simulink model "SIMULINK_ADP_Tracking"  (R2023b)
settings: Solver=FixedStepAuto  StartTime=0.0  StopTime=sim_end_time  FixedStep=fixed_step_size  RelTol=1e-3
undefined symbols (not defined in the file): a, act_end, b, battery_threshold, bb, delta_, draw_gif, droneyeeUAV2_NUM, droneyeeUAV3_NUM, droneyeeUAV4_NUM, droneyeeUAV5_NUM, fixed_step_size, k, KD_x, KD_y, kd_z, KDD_x, KDD_y, KI_x, KI_y, ki_z, KII_x, KII_y, KP_x, KP_y, kp_z, KPP_x, KPP_y, lmt, omega, omega_, R, sim_end_time, uav10num, uav1num, uav2num, uav3num, uav4num, uav5num, uav6num, uav7num, uav8num, uav9num, UAV_NUM, Vel_Switch_1, Vel_Switch_10, Vel_Switch_11, Vel_Switch_12, Vel_Switch_13, Vel_Switch_14, Vel_Switch_15, Vel_Switch_16, Vel_Switch_17, Vel_Switch_18, Vel_Switch_19, Vel_Switch_2, Vel_Switch_20, Vel_Switch_3, Vel_Switch_4, Vel_Switch_5 ... (+16)
libraries: simulink x118, aerolibanimutils x1
(part 1 of 11)
settings Model: Creator=exbot  LastModifiedBy=tanju
settings SolverCC: AlgebraicLoopSolver=TrustRegion
settings DataIOCC: LimitDataPoints=on  ReturnWorkspaceOutputs=off
settings OptimizationCC: DefaultParameterBehavior=Inlined  ReuseModelBlockBuffer=off  PassReuseOutputArgsAs=Individual arguments  MaxStackSize=64  EfficientTunableParamExpr=on
settings DebuggingCC: ParameterTunabilityLossMsg=error  UnconnectedInputMsg=warning  UnconnectedOutputMsg=warning  UnconnectedLineMsg=warning  AllowSymbolicDim=off  SFUnexpectedBacktrackingDiag=warning  SFNoUnconditionalDefaultTransitionDiag=warning  SFExecutionAtInitializationDiag=none  ArithmeticOperatorsInVariantConditions=warning
settings HardwareCC: ProdBitPerPointer=32  ProdBitPerSizeT=32  ProdBitPerPtrDiffT=32  ProdLargestAtomicFloat=None  ProdIntDivRoundTo=Undefined  ProdEndianess=Unspecified  ProdWordSize=32  ProdHWDeviceType=Generic->Unspecified (assume 32-bit Generic)  TargetBitPerPointer=64  TargetBitPerSizeT=64  TargetBitPerPtrDiffT=64  TargetLongLongMode=on  TargetIntDivRoundTo=Zero  TargetEndianess=LittleEndian  TargetWordSize=64  TargetHWDeviceType=MATLAB Host  ProdEqTarget=off
settings ModelReferenceCC: EnableRefExpFcnMdlSchedulingChecks=on  PropagateSignalLabelsOutOfModel=off
settings SFSimCC: SimUseLocalCustomCode=off  MATLABDynamicMemAlloc=off  CustomCodeUndefinedFunction=UseInterfaceOnly
settings RTWCC: Description=Embedded Coder (host-based shared library target)  SystemTargetFile=ert_shrlib.tlc  TemplateMakefile=ert_default_tmf  GenerateReport=on  RTWUseLocalCustomCode=off  IncludeHyperlinkInReport=on  LaunchReport=on  GenerateTraceInfo=on  GenerateTraceReport=on  GenerateTraceReportSl=on  GenerateTraceReportSf=on  GenerateTraceReportEml=on
settings CodeAppCC: ForceParamTrailComments=on  IgnoreCustomStorageClasses=off  OperatorAnnotations=on  SimulinkDataObjDesc=on  SFDataObjDesc=on  InsertBlockDesc=on
settings STFCustomTargetCC: TargetLangStandard=C89/C90 (ANSI)  MultiwordLength=256  GenerateSampleERTMain=on  ParMdlRefBuildCompliant=on  CompOptLevelCompliant=on  CombineOutputUpdateFcns=on  ERTCustomFileBanners=on  RemoveResetFunc=on  MATLABClassNameForMDSCustomization=Simulink.SoftwareTarget.ERTCustomization  ModelStepFunctionPrototypeControlCompliant=on  UseToolchainInfoCompliant=on  SystemTargetFile=ert_shrlib.tlc
settings ERTTargetCC: GenerateSampleERTMain=on  ConcurrentExecutionCompliant=off  SupportContinuousTime=on  SupportNonInlinedSFcns=on  CPPClassGenCompliant=off  InlinedParameterPlacement=NonHierarchical  ERTCustomFileTemplate=example_file_process.tlc
settings ConfigComp: CovMetricSettings=dw  CovSaveCumulativeToWorkspaceVar=on  CovSaveSingleToWorkspaceVar=on  CovExternalEMLEnable=off

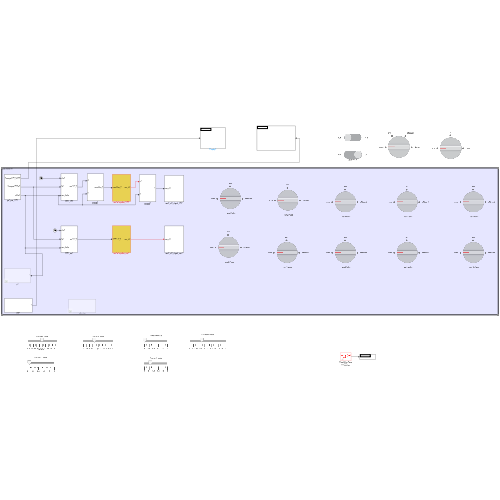
[thumbnail: Simulink's stored preview of the top-level diagram]
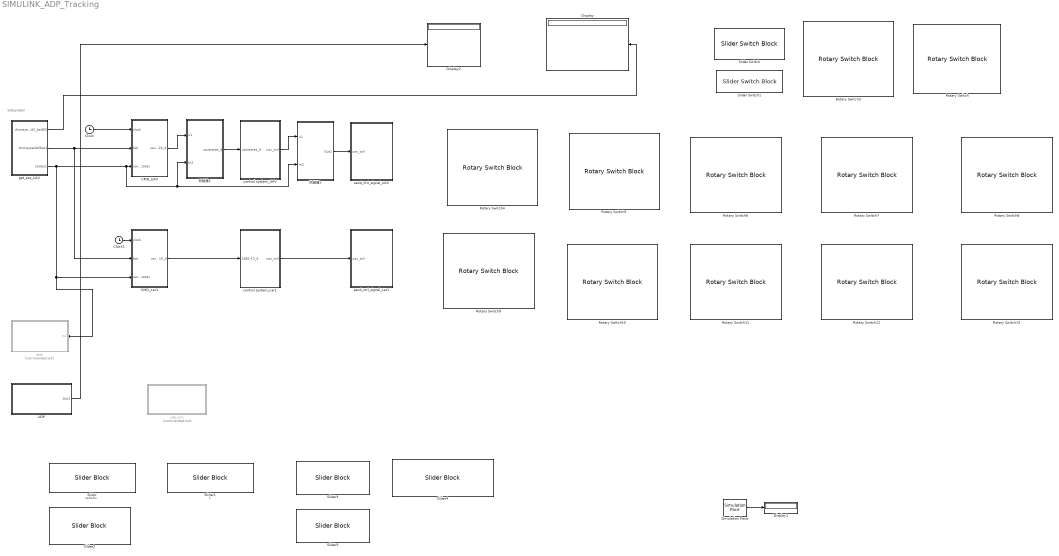
== system SIMULINK_ADP_Tracking ==
  note: Subsystem
  note: safedis
  note: k
  CMD_UAV : Subsystem
  CMD_car1 : Subsystem
  Clock : Clock
  Clock1 : Clock
  Display : Display
  Display1 : Display
  Display2 : Display
  Rotary Switch : RotarySwitchBlock  LabelPosition=Hide
      settings: Values={{'land', 'trj', 'hover'}, [-1 2 1]}
  Rotary Switch{4..13} (10 alike) : RotarySwitchBlock  LabelPosition=Bottom
      settings: Values={{'none', 'arm', 'offboard'}, [0 2 3]}
  Rotary Switch3 : RotarySwitchBlock  LabelPosition=Hide
      settings: Values={{'none', 'arm', 'offboard', 'disram'}, [0 2 3 5]}
  Simulation Pace : aerolibanimutils/Simulation Pace  SimulationPace=1  SleepMode=MATLAB Thread  OutputPaceError=on  SampleTime=-1
  Slider{,2..5} (5 alike) : SliderBlock  ScaleMax=2
  Slider Switch : SliderSwitchBlock  LabelPosition=Hide
      settings: Values={{'仿真', '实飞'}, [-1 1]}
  Slider Switch1 : SliderSwitchBlock  LabelPosition=Bottom
      settings: Values={{'Off', 'On'}, [0 1]}
  Slider1 : SliderBlock  ScaleMax=5
  UDP : Subsystem
  control system_UAV : Subsystem
  control system_car1 : Subsystem
  get_pos_UAV : Subsystem
  plot : Subsystem  Commented=on
  send_ctrl_signal_UAV : Subsystem
  send_ctrl_signal_car1 : Subsystem
  udp_sim : Subsystem  Commented=on
  防碰撞1 : Subsystem
  防碰撞2 : Subsystem
  wires:
  Simulation Pace/1 -> Display1/1
  UDP/1(Out1) -> Display2/1
  get_pos_UAV/1(droneyeeUAV_batDIS) -> Display/1
  防碰撞1/1(uavstates_d) -> control system_UAV/1(uavstates_d)
  CMD_UAV/1(uav1-24_d) -> 防碰撞1/1(u1)
  control system_UAV/1(uav_ctrl) -> 防碰撞2/1(u1)
  防碰撞2/1(Out1) -> send_ctrl_signal_UAV/1(uav_ctrl)
  Clock1/1 -> CMD_car1/1(clock)
  get_pos_UAV/3(states1) -> CMD_car1/3(uav_states), plot/1(In1), 防碰撞2/2(In2), 防碰撞1/2(In2), CMD_UAV/3(uav_states)
  Clock/1 -> CMD_UAV/1(clock)
  get_pos_UAV/2(droneyeeUAVbat1) -> CMD_car1/2(bat), CMD_UAV/2(bat)
  control system_car1/1(uav_ctrl) -> send_ctrl_signal_car1/1(uav_ctrl)
  CMD_car1/1(car1-10_d) -> control system_car1/1(CAR1-10_d)

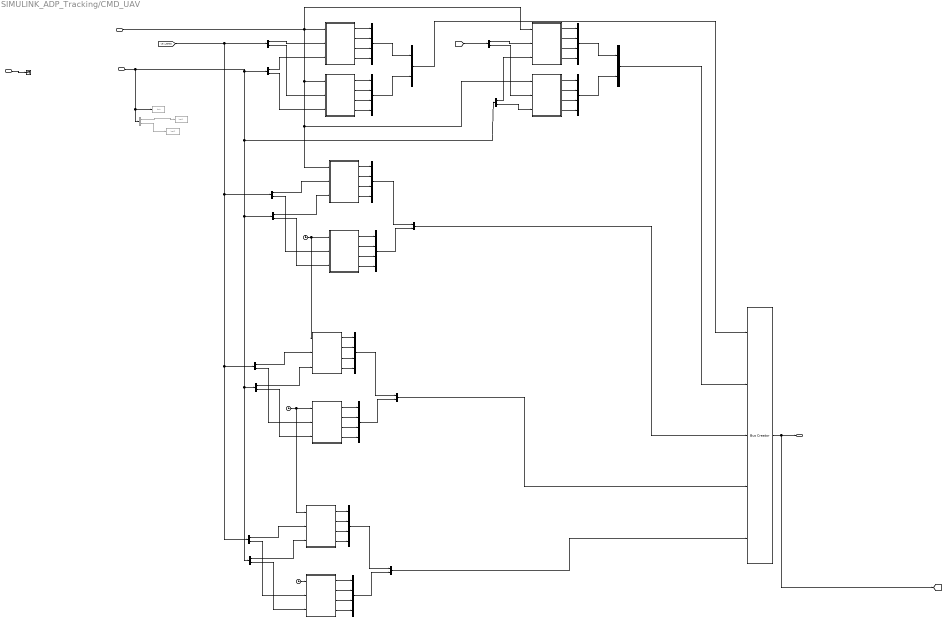
== system SIMULINK_ADP_Tracking/CMD_UAV ==
  clock : Inport
  bat : Inport  Port=2
  uav_states : Inport  Port=3
  Bus Creator{,1,3..4,6..7,9..10,12..13} (10 alike) : BusCreator  Inputs=4
  Bus Creator{2,5,8,11,14} (5 alike) : BusCreator  Inputs=2
  Bus Creator36 : BusCreator  Inputs=5
  Bus Selector : BusSelector  OutputSignals=droneyeeUAV1bat,droneyeeUAV2bat
  Bus Selector1 : BusSelector  OutputSignals=droneyeeUAV1_states,droneyeeUAV2_states
  Bus Selector10 : BusSelector  OutputSignals=droneyeeUAV9bat,droneyeeUAV10bat
  Bus Selector2 : BusSelector  OutputSignals=droneyeeUAV5_states,droneyeeUAV6_states
  Bus Selector3 : BusSelector  OutputSignals=droneyeeUAV3_states,droneyeeUAV4_states
  Bus Selector4 : BusSelector  OutputSignals=droneyeeUAV3bat,droneyeeUAV4bat
  Bus Selector5 : BusSelector  OutputSignals=droneyeeUAV5bat,droneyeeUAV6bat
  Bus Selector6 : BusSelector  Commented=on  OutputSignals=droneyeeUAV1bat,droneyeeUAV2bat
  Bus Selector7 : BusSelector  OutputSignals=droneyeeUAV7_states,droneyeeUAV8_states
  Bus Selector8 : BusSelector  OutputSignals=droneyeeUAV7bat,droneyeeUAV8bat
  Bus Selector9 : BusSelector  OutputSignals=droneyeeUAV9_states,droneyeeUAV10_states
  CMD1 : Subsystem
  CMD10 : Subsystem
  CMD2 : Subsystem
  CMD3 : Subsystem
  CMD4 : Subsystem
  CMD5 : Subsystem
  CMD6 : Subsystem
  CMD7 : Subsystem
  CMD8 : Subsystem
  CMD9 : Subsystem
  Clock : Clock
  Clock1 : Clock
  Clock2 : Clock
  Terminator : Terminator
  To Workspace : ToWorkspace  Commented=on  VariableName=bat  SampleTime=-1
  To Workspace1 : ToWorkspace  Commented=on  VariableName=bat1  SampleTime=-1
  To Workspace2 : ToWorkspace  Commented=on  VariableName=bat2  SampleTime=-1
  uav1-24_d : Outport  VectorParamsAs1DForOutWhenUnconnected=off
  tag scope: uav1_24_d1=global
  wires:
  CMD1/1(x_d) -> Bus Creator/1  "x1_d"
  CMD1/2(y_d) -> Bus Creator/2  "y1_d"
  CMD1/3(z_d) -> Bus Creator/3  "z1_d"
  CMD1/4(yaw_d) -> Bus Creator/4  "yaw1_d"
  CMD2/1(x_d) -> Bus Creator1/1  "x2_d"
  CMD2/2(y_d) -> Bus Creator1/2  "y2_d"
  CMD2/3(z_d) -> Bus Creator1/3  "z2_d"
  CMD2/4(yaw_d) -> Bus Creator1/4  "yaw2_d"
  Bus Creator/1 -> Bus Creator2/1  "droneyeeUAV1_d"
  Bus Creator1/1 -> Bus Creator2/2  "droneyeeUAV2_d"
  Bus Creator2/1 -> Bus Creator36/1  "states1_2_d"
  Bus Creator3/1 -> Bus Creator5/1  "droneyeeUAV3_d"
  Bus Creator4/1 -> Bus Creator5/2  "droneyeeUAV4_d"
  CMD3/2(y_d) -> Bus Creator3/2  "y3_d"
  CMD3/3(z_d) -> Bus Creator3/3  "z3_d"
  CMD3/4(yaw_d) -> Bus Creator3/4  "yaw3_d"
  Bus Creator5/1 -> Bus Creator36/2  "states_3_4_d"
  CMD4/1(x_d) -> Bus Creator4/1  "x4_d"
  CMD3/1(x_d) -> Bus Creator3/1  "x3_d"
  CMD4/2(y_d) -> Bus Creator4/2  "y4_d"
  CMD4/4(yaw_d) -> Bus Creator4/4  "yaw4_d"
  CMD4/3(z_d) -> Bus Creator4/3  "z4_d"
  CMD5/2(y_d) -> Bus Creator6/2  "y5_d"
  CMD5/3(z_d) -> Bus Creator6/3  "z5_d"
  CMD5/4(yaw_d) -> Bus Creator6/4  "yaw5_d"
  CMD5/1(x_d) -> Bus Creator6/1  "x5_d"
  Bus Creator8/1 -> Bus Creator36/3  "states_5_6_d"
  Bus Selector1/1 -> CMD1/2(droneyeeUAV_states)  "<droneyeeUAV1_states>"
  Bus Selector1/2 -> CMD2/2(droneyeeUAV_states)  "<droneyeeUAV2_states>"
  Bus Selector/1 -> CMD1/3(droneyeeUAV_bat)  "<droneyeeUAV1bat>"
  Bus Selector/2 -> CMD2/3(droneyeeUAV_bat)  "<droneyeeUAV2bat>"
  Bus Selector2/1 -> CMD5/2(droneyeeUAV_states)  "<droneyeeUAV5_states>"
  [uav_states] -> Bus Selector3/1
  Bus Selector3/1 -> CMD3/2(droneyeeUAV_states)  "<droneyeeUAV3_states>"
  Bus Selector3/2 -> CMD4/2(droneyeeUAV_states)  "<droneyeeUAV4_states>"
  Bus Selector4/1 -> CMD3/3(droneyeeUAV_bat)  "<droneyeeUAV3bat>"
  Bus Selector4/2 -> CMD4/3(droneyeeUAV_bat)  "<droneyeeUAV4bat>"
  Bus Selector5/1 -> CMD5/3(droneyeeUAV_bat)  "<droneyeeUAV5bat>"
  clock/1 -> CMD3/1("clock "), CMD2/1("clock "), CMD4/1("clock "), CMD5/1("clock "), CMD1/1("clock ")
  Bus Creator36/1 -> [uav1_24_d1], uav1-24_d/1
  uav_states/1 -> Terminator/1
  Bus Selector6/1 -> To Workspace1/1  "<droneyeeUAV1bat>"
  Bus Selector6/2 -> To Workspace2/1  "<droneyeeUAV2bat>"
  CMD6/2(y_d) -> Bus Creator7/2  "y1_d"
  CMD6/1(x_d) -> Bus Creator7/1  "x1_d"
  CMD6/3(z_d) -> Bus Creator7/3  "z1_d"
  CMD6/4(yaw_d) -> Bus Creator7/4  "yaw1_d"
  Bus Selector5/2 -> CMD6/3(droneyeeUAV_bat)  "<droneyeeUAV6bat>"
  Bus Selector2/2 -> CMD6/2(droneyeeUAV_states)  "<droneyeeUAV6_states>"
  Bus Creator6/1 -> Bus Creator8/1  "droneyeeUAV5_d"
  Bus Creator7/1 -> Bus Creator8/2  "droneyeeUAV4_d"
  Bus Creator10/1 -> Bus Creator11/2  "droneyeeUAV4_d"
  Clock/1 -> CMD7/1("clock "), CMD6/1("clock ")
  CMD7/1(x_d) -> Bus Creator9/1  "x5_d"
  Bus Creator9/1 -> Bus Creator11/1  "droneyeeUAV5_d"
  Bus Selector7/1 -> CMD7/2(droneyeeUAV_states)  "<droneyeeUAV7_states>"
  CMD7/4(yaw_d) -> Bus Creator9/4  "yaw5_d"
  Bus Selector8/1 -> CMD7/3(droneyeeUAV_bat)  "<droneyeeUAV7bat>"
  CMD7/2(y_d) -> Bus Creator9/2  "y5_d"
  CMD7/3(z_d) -> Bus Creator9/3  "z5_d"
  CMD8/2(y_d) -> Bus Creator10/2  "y1_d"
  CMD8/3(z_d) -> Bus Creator10/3  "z1_d"
  CMD8/1(x_d) -> Bus Creator10/1  "x1_d"
  Bus Selector8/2 -> CMD8/3(droneyeeUAV_bat)  "<droneyeeUAV8bat>"
  Bus Selector7/2 -> CMD8/2(droneyeeUAV_states)  "<droneyeeUAV8_states>"
  CMD8/4(yaw_d) -> Bus Creator10/4  "yaw1_d"
  Bus Creator13/1 -> Bus Creator14/2  "droneyeeUAV4_d"
  Clock1/1 -> CMD8/1("clock "), CMD9/1("clock ")
  CMD9/1(x_d) -> Bus Creator12/1  "x5_d"
  Bus Creator12/1 -> Bus Creator14/1  "droneyeeUAV5_d"
  bat/1 -> Bus Selector6/1, To Workspace/1, Bus Selector10/1, Bus Selector8/1, Bus Selector5/1, Bus Selector4/1, Bus Selector/1
  Bus Selector9/1 -> CMD9/2(droneyeeUAV_states)  "<droneyeeUAV9_states>"
  CMD9/4(yaw_d) -> Bus Creator12/4  "yaw5_d"
  [uav_states] -> Bus Selector9/1, Bus Selector7/1, Bus Selector2/1, Bus Selector1/1
  Bus Selector10/1 -> CMD9/3(droneyeeUAV_bat)  "<droneyeeUAV9bat>"
  CMD9/2(y_d) -> Bus Creator12/2  "y5_d"
  CMD9/3(z_d) -> Bus Creator12/3  "z5_d"
  CMD10/2(y_d) -> Bus Creator13/2  "y1_d"
  CMD10/3(z_d) -> Bus Creator13/3  "z1_d"
  CMD10/1(x_d) -> Bus Creator13/1  "x1_d"
  Bus Selector10/2 -> CMD10/3(droneyeeUAV_bat)  "<droneyeeUAV10bat>"
  Clock2/1 -> CMD10/1("clock ")
  Bus Selector9/2 -> CMD10/2(droneyeeUAV_states)  "<droneyeeUAV10_states>"
  CMD10/4(yaw_d) -> Bus Creator13/4  "yaw1_d"
  Bus Creator11/1 -> Bus Creator36/4  "states_7_8_d"
  Bus Creator14/1 -> Bus Creator36/5  "states_9_10_d"

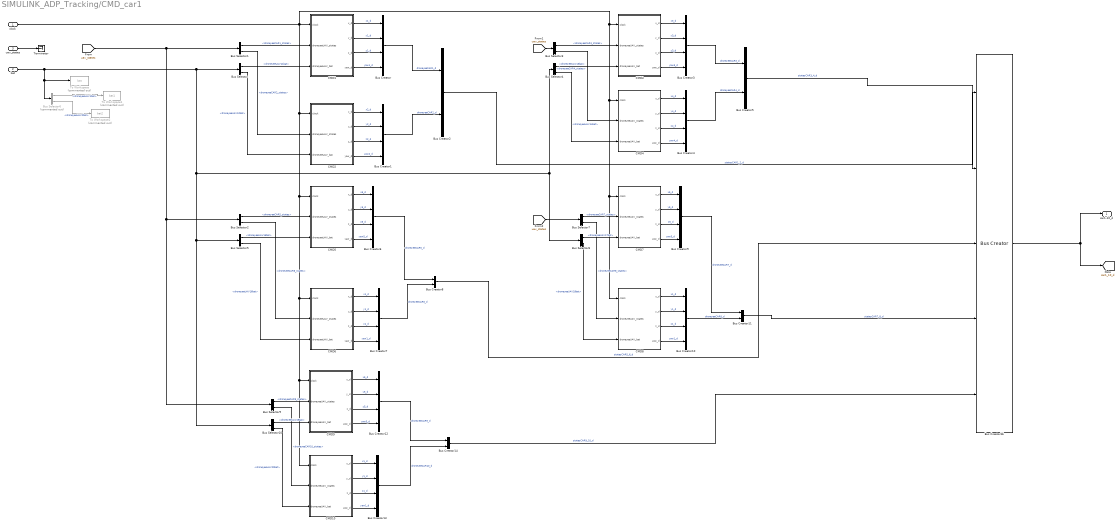
== system SIMULINK_ADP_Tracking/CMD_car1 ==
  clock : Inport
  bat : Inport  Port=2
  uav_states : Inport  Port=3
  Bus Creator{,1,3..4,6..7,9..10,12..13} (10 alike) : BusCreator  Inputs=4
  Bus Creator{2,5,8,11,14} (5 alike) : BusCreator  Inputs=2
  Bus Creator36 : BusCreator  Inputs=5
  Bus Selector : BusSelector  OutputSignals=droneyeeUAV11bat,droneyeeUAV12bat
  Bus Selector1 : BusSelector  OutputSignals=droneyeeCAR1_states,droneyeeCAR2_states
  Bus Selector10 : BusSelector  OutputSignals=droneyeeUAV19bat,droneyeeUAV20bat
  Bus Selector2 : BusSelector  OutputSignals=droneyeeCAR5_states,droneyeeCAR6_states
  Bus Selector3 : BusSelector  OutputSignals=droneyeeCAR3_states,droneyeeCAR4_states
  Bus Selector4 : BusSelector  OutputSignals=droneyeeUAV13bat,droneyeeUAV14bat
  Bus Selector5 : BusSelector  OutputSignals=droneyeeUAV15bat,droneyeeUAV16bat
  Bus Selector6 : BusSelector  Commented=on  OutputSignals=droneyeeUAV1bat,droneyeeUAV2bat
  Bus Selector7 : BusSelector  OutputSignals=droneyeeCAR7_states,droneyeeCAR8_states
  Bus Selector8 : BusSelector  OutputSignals=droneyeeUAV17bat,droneyeeUAV18bat
  Bus Selector9 : BusSelector  OutputSignals=droneyeeCAR9_states,droneyeeCAR10_states
  CMD1 : Subsystem
  CMD10 : Subsystem
  CMD2 : Subsystem
  CMD3 : Subsystem
  CMD4 : Subsystem
  CMD5 : Subsystem
  CMD6 : Subsystem
  CMD7 : Subsystem
  CMD8 : Subsystem
  CMD9 : Subsystem
  Terminator : Terminator
  To Workspace : ToWorkspace  Commented=on  VariableName=bat  SampleTime=-1
  To Workspace1 : ToWorkspace  Commented=on  VariableName=bat1  SampleTime=-1
  To Workspace2 : ToWorkspace  Commented=on  VariableName=bat2  SampleTime=-1
  car1-10_d : Outport  VectorParamsAs1DForOutWhenUnconnected=off
  tag scope: car1_10_d=global
  wires:
  CMD1/1(x_d) -> Bus Creator/1  "x1_d"
  CMD1/2(y_d) -> Bus Creator/2  "y1_d"
  CMD1/3(z_d) -> Bus Creator/3  "z1_d"
  CMD1/4(yaw_d) -> Bus Creator/4  "yaw1_d"
  CMD2/1(x_d) -> Bus Creator1/1  "x2_d"
  CMD2/2(y_d) -> Bus Creator1/2  "y2_d"
  CMD2/3(z_d) -> Bus Creator1/3  "z2_d"
  CMD2/4(yaw_d) -> Bus Creator1/4  "yaw2_d"
  Bus Creator/1 -> Bus Creator2/1  "droneyeeCAR1_d"
  Bus Creator1/1 -> Bus Creator2/2  "droneyeeCAR2_d"
  Bus Creator3/1 -> Bus Creator5/1  "droneyeeCAR3_d"
  Bus Creator4/1 -> Bus Creator5/2  "droneyeeCAR4_d"
  CMD3/2(y_d) -> Bus Creator3/2  "y3_d"
  CMD3/3(z_d) -> Bus Creator3/3  "z3_d"
  CMD3/4(yaw_d) -> Bus Creator3/4  "yaw3_d"
  Bus Creator5/1 -> Bus Creator36/2  "statesCAR3_4_d"
  CMD4/1(x_d) -> Bus Creator4/1  "x4_d"
  CMD3/1(x_d) -> Bus Creator3/1  "x3_d"
  CMD4/2(y_d) -> Bus Creator4/2  "y4_d"
  CMD4/4(yaw_d) -> Bus Creator4/4  "yaw4_d"
  CMD4/3(z_d) -> Bus Creator4/3  "z4_d"
  CMD5/2(y_d) -> Bus Creator6/2  "y5_d"
  CMD5/3(z_d) -> Bus Creator6/3  "z5_d"
  CMD5/4(yaw_d) -> Bus Creator6/4  "yaw5_d"
  CMD5/1(x_d) -> Bus Creator6/1  "x5_d"
  Bus Creator8/1 -> Bus Creator36/3  "statesCAR5_6_d"
  Bus Selector1/1 -> CMD1/2(droneyeeUAV_states)  "<droneyeeCAR1_states>"
  Bus Selector1/2 -> CMD2/2(droneyeeUAV_states)  "<droneyeeCAR2_states>"
  Bus Selector/1 -> CMD1/3(droneyeeUAV_bat)  "<droneyeeUAV11bat>"
  Bus Selector/2 -> CMD2/3(droneyeeUAV_bat)  "<droneyeeUAV12bat>"
  Bus Selector2/1 -> CMD5/2(droneyeeUAV_states)  "<droneyeeCAR5_states>"
  [uav_states] -> Bus Selector3/1
  Bus Selector3/1 -> CMD3/2(droneyeeUAV_states)  "<droneyeeCAR3_states>"
  Bus Selector3/2 -> CMD4/2(droneyeeUAV_states)  "<droneyeeCAR4_states>"
  Bus Selector4/1 -> CMD3/3(droneyeeUAV_bat)  "<droneyeeUAV13bat>"
  Bus Selector4/2 -> CMD4/3(droneyeeUAV_bat)  "<droneyeeUAV14bat>"
  Bus Selector5/1 -> CMD5/3(droneyeeUAV_bat)  "<droneyeeUAV15bat>"
  clock/1 -> CMD8/1("clock "), CMD7/1("clock "), CMD4/1("clock "), CMD3/1("clock "), CMD10/1("clock "), CMD9/1("clock "), CMD6/1("clock "), CMD5/1("clock "), CMD2/1("clock "), CMD1/1("clock ")
  Bus Creator36/1 -> car1-10_d/1, [car1_10_d]
  uav_states/1 -> Terminator/1
  Bus Selector6/1 -> To Workspace1/1  "<droneyeeUAV1bat>"
  Bus Selector6/2 -> To Workspace2/1  "<droneyeeUAV2bat>"
  CMD6/2(y_d) -> Bus Creator7/2  "y1_d"
  CMD6/1(x_d) -> Bus Creator7/1  "x1_d"
  CMD6/3(z_d) -> Bus Creator7/3  "z1_d"
  CMD6/4(yaw_d) -> Bus Creator7/4  "yaw1_d"
  Bus Selector5/2 -> CMD6/3(droneyeeUAV_bat)  "<droneyeeUAV16bat>"
  Bus Selector2/2 -> CMD6/2(droneyeeUAV_states)  "<droneyeeCAR6_states>"
  Bus Creator6/1 -> Bus Creator8/1  "droneyeeCAR5_d"
  Bus Creator7/1 -> Bus Creator8/2  "droneyeeCAR6_d"
  Bus Creator10/1 -> Bus Creator11/2  "droneyeeCAR8_d"
  CMD7/1(x_d) -> Bus Creator9/1  "x5_d"
  Bus Creator9/1 -> Bus Creator11/1  "droneyeeCAR7_d"
  Bus Selector7/1 -> CMD7/2(droneyeeUAV_states)  "<droneyeeCAR7_states>"
  CMD7/4(yaw_d) -> Bus Creator9/4  "yaw5_d"
  Bus Selector8/1 -> CMD7/3(droneyeeUAV_bat)  "<droneyeeUAV17bat>"
  CMD7/2(y_d) -> Bus Creator9/2  "y5_d"
  CMD7/3(z_d) -> Bus Creator9/3  "z5_d"
  CMD8/2(y_d) -> Bus Creator10/2  "y1_d"
  CMD8/3(z_d) -> Bus Creator10/3  "z1_d"
  CMD8/1(x_d) -> Bus Creator10/1  "x1_d"
  Bus Selector8/2 -> CMD8/3(droneyeeUAV_bat)  "<droneyeeUAV18bat>"
  Bus Selector7/2 -> CMD8/2(droneyeeUAV_states)  "<droneyeeCAR8_states>"
  CMD8/4(yaw_d) -> Bus Creator10/4  "yaw1_d"
  Bus Creator13/1 -> Bus Creator14/2  "droneyeeCAR10_d"
  CMD9/1(x_d) -> Bus Creator12/1  "x5_d"
  Bus Creator12/1 -> Bus Creator14/1  "droneyeeCAR9_d"
  bat/1 -> Bus Selector6/1, To Workspace/1, Bus Selector10/1, Bus Selector5/1, Bus Selector8/1, Bus Selector4/1, Bus Selector/1
  CMD9/4(yaw_d) -> Bus Creator12/4  "yaw5_d"
  [uav_states] -> Bus Selector9/1, Bus Selector2/1, Bus Selector1/1
  CMD9/2(y_d) -> Bus Creator12/2  "y5_d"
  CMD9/3(z_d) -> Bus Creator12/3  "z5_d"
  CMD10/2(y_d) -> Bus Creator13/2  "y1_d"
  CMD10/3(z_d) -> Bus Creator13/3  "z1_d"
  CMD10/1(x_d) -> Bus Creator13/1  "x1_d"
  CMD10/4(yaw_d) -> Bus Creator13/4  "yaw1_d"
  Bus Creator11/1 -> Bus Creator36/4  "statesCAR7_8_d"
  Bus Creator14/1 -> Bus Creator36/5  "statesCAR9_10_d"
  [uav_states] -> Bus Selector7/1
  Bus Selector9/1 -> CMD9/2(droneyeeUAV_states)  "<droneyeeCAR9_states>"
  Bus Selector9/2 -> CMD10/2(droneyeeUAV_states)  "<droneyeeCAR10_states>"
  Bus Selector10/1 -> CMD9/3(droneyeeUAV_bat)  "<droneyeeUAV19bat>"
  Bus Selector10/2 -> CMD10/3(droneyeeUAV_bat)  "<droneyeeUAV20bat>"
  Bus Creator2/1 -> Bus Creator36/1  "statesCAR1_2_d"

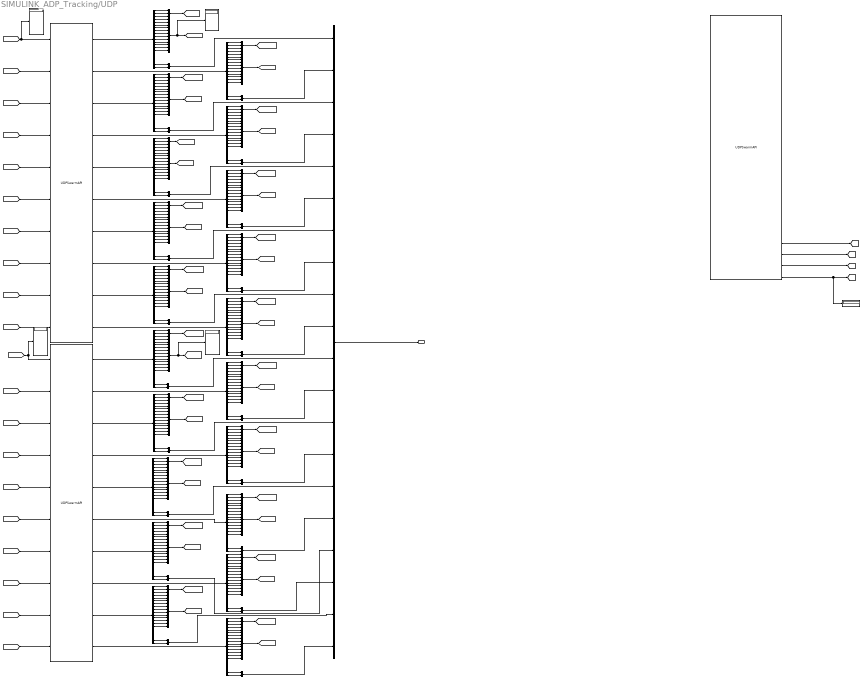
== system SIMULINK_ADP_Tracking/UDP ==
  note: 这个UDP模块的端口为 26000+(Id-1)*2
      | Simulink输入维度为0,
      | 输出维度为3，对应UDP接收的[Double bat1, Double bat2, Double bat3]
      |
      | 这个UDP模块的发送端口为 26000+(Id-1)*2+1（但是这里没有使用）
  CopterRecA : S-Function  FunctionName=UDPSwarmAPI  Parameters=port,num,modeValue,T,ip  SFunctionDeploymentMode=off  EnableBusSupport=off  mask(UDP Receive){ip=127.0.0.1, port=27000, num=10, mode=CopterRecA, T=-1, modeValue=0}
      mask prompts: ip "UDP IP Address"; port "UDP Port"; num "vehicle Number"; mode "UDP Mode"; T "Sample Time"
      mask help:
      | This block receives bytes from an UDP/IP connection.
      | The first parameter is the UDP port on the first CopterSim App
      | The second parameter is the total vehicle number
      | The third parameter is the data mode. check the help button for the definition
      mask init:
      | if strcmp(mode,'CopterRecA')
      |     modeValue = 0;
      | elseif strcmp(mode,'CopterRecB') 
      |     modeValue = 1;
      | else
      |     modeValue = 0;
      | end
      mask Help:
      | UDP mode = 0 (localhost) or 1(broadcast), the 28-D output is defined as:
      | for(int i=0;i<3;i++){
      |     data[0+i]=(double)stl.gpsHome[i];
      |     data[3+i]=(double)stl.AngEular[i];
      |     data[6+i]=(double)stl.localPos[i];
      |     data[9+i]=(double)stl.localVel[i];
      |     data[12+i]=(double)stl.GpsPos[i];
      |     data[15+i]=(double)stl.GpsVel[i];
      | }
      | data[18] = (double)stl.time_boot_ms;
      | data[19] = (double)stl.copterID;
      | data[20] = (double)stl.relative_alt;
      | data[21] = (double)stl.hdg;
      | data[22] = (double)stl.satellites_visible;
      | data[23] = (double)stl.fix_type;
      | data[24] = (double)stl.resrveInit;
      | data[25] = (double)stl.pos_horiz_accuracy;
      | data[26] = (double)stl.pos_vert_accuracy;
      | data[27] = (double)stl.resrveFloat;
      | 
      | UDP mode =  2 (localhost) or 3(broadcast), 4,5 the 12-D output is defined as:
      | 
      | if(iUdpMode==2||iUdpMode==3){
      |     for(int i=0;i<3;i++){
      |         data[i]=(double)st.gpsHome[i];
      |         data[i+3]=(double)st.AngEular[i];
      |         data[i+6]=(double)st.localPos[i];
      |         data[i+9]=(double)st.localVel[i];
      |     }
      | }
      | if(iUdpMode==4||iUdpMode==5){
      |     double GpsHomePos[3];
      |     for(int i=0;i<3;i++){
      |             GpsHomePos[i] = (double)st.gpsHome[i];
      |             data[3+i]=(double)st.localPos[i];
      |             data[6+i]=(double)st.localVel[i];
      |             data[9+i]=(double)st.AngEular[i];
      |     }
      |     double PIR = 3.1415926536;
      |     data[0]=(GpsHomePos[0]*1e-7-40.1540302)/180*PIR*6362000+(double)st.localPos[0];
      |     data[1]=(GpsHomePos[1]*1e-7-116.2593683)/180*PIR*6362000+(double)st.localPos[1];
      |     data[2]=-GpsHomePos[2]*1e-3+(double)st.localPos[2];
      | }
      | 
      | The above structure is
      | struct outHILStateData{ // mavlink data forward from Pixhawk
      |     uint32_t time_boot_ms; //Timestamp of the message
      |     uint32_t copterID;     //Copter ID start from 1
      |     int32_t GpsPos[3];     //Estimated GPS position，lat&long: deg*1e7, alt: m*1e3 and up is positive
      |     int32_t GpsVel[3];     //Estimated GPS velocity, NED, m/s*1e2->cm/s
      |     int32_t gpsHome[3];     //Home GPS position, lat&long: deg*1e7, alt: m*1e3 and up is positive
      |     int32_t relative_alt;  //alt: m*1e3 and up is positive
      |     int32_t hdg;           //Course angle, NED,deg*1000, 0~360
      |     int32_t satellites_visible; //GPS Raw data, sum of satellite
      |     int32_t fix_type;     //GPS Raw data, Fixed type, 3 for fixed (good precision)
      |     int32_t resrveInit;       //Int, reserve for the future use
      |     float AngEular[3];    //Estimated Euler angle, unit: rad/s
      |     float localPos[3];    //Estimated locoal position, NED, unit: m
      |     float localVel[3];    //Estimated locoal velocity, NED, unit: m/s
      |     float pos_horiz_accuracy;   //GPS horizontal accuracy, unit: m
      |     float pos_vert_accuracy; //GPS vertical accuracy, unit: m
      |     float resrveFloat;      //float,reserve for the future use
      | }
      mask TypeOptions mode: CopterRecA | CopterRecB
  CopterRecA1 : S-Function  FunctionName=UDPSwarmAPI  Parameters=port,num,modeValue,T,ip  SFunctionDeploymentMode=off  EnableBusSupport=off  mask(UDP Receive){ip=127.0.0.1, port=28000, num=10, mode=CopterRecA, T=-1, modeValue=0}
      mask prompts: ip "UDP IP Address"; port "UDP Port"; num "vehicle Number"; mode "UDP Mode"; T "Sample Time"
      mask help:
      | This block receives bytes from an UDP/IP connection.
      | The first parameter is the UDP port on the first CopterSim App
      | The second parameter is the total vehicle number
      | The third parameter is the data mode. check the help button for the definition
      mask init:
      | if strcmp(mode,'CopterRecA')
      |     modeValue = 0;
      | elseif strcmp(mode,'CopterRecB') 
      |     modeValue = 1;
      | else
      |     modeValue = 0;
      | end
      mask Help:
      | UDP mode = 0 (localhost) or 1(broadcast), the 28-D output is defined as:
      | for(int i=0;i<3;i++){
      |     data[0+i]=(double)stl.gpsHome[i];
      |     data[3+i]=(double)stl.AngEular[i];
      |     data[6+i]=(double)stl.localPos[i];
      |     data[9+i]=(double)stl.localVel[i];
      |     data[12+i]=(double)stl.GpsPos[i];
      |     data[15+i]=(double)stl.GpsVel[i];
      | }
      | data[18] = (double)stl.time_boot_ms;
      | data[19] = (double)stl.copterID;
      | data[20] = (double)stl.relative_alt;
      | data[21] = (double)stl.hdg;
      | data[22] = (double)stl.satellites_visible;
      | data[23] = (double)stl.fix_type;
      | data[24] = (double)stl.resrveInit;
      | data[25] = (double)stl.pos_horiz_accuracy;
      | data[26] = (double)stl.pos_vert_accuracy;
      | data[27] = (double)stl.resrveFloat;
      | 
      | UDP mode =  2 (localhost) or 3(broadcast), 4,5 the 12-D output is defined as:
      | 
      | if(iUdpMode==2||iUdpMode==3){
      |     for(int i=0;i<3;i++){
      |         data[i]=(double)st.gpsHome[i];
      |         data[i+3]=(double)st.AngEular[i];
      |         data[i+6]=(double)st.localPos[i];
      |         data[i+9]=(double)st.localVel[i];
      |     }
      | }
      | if(iUdpMode==4||iUdpMode==5){
      |     double GpsHomePos[3];
      |     for(int i=0;i<3;i++){
      |             GpsHomePos[i] = (double)st.gpsHome[i];
      |             data[3+i]=(double)st.localPos[i];
      |             data[6+i]=(double)st.localVel[i];
      |             data[9+i]=(double)st.AngEular[i];
      |     }
      |     double PIR = 3.1415926536;
      |     data[0]=(GpsHomePos[0]*1e-7-40.1540302)/180*PIR*6362000+(double)st.localPos[0];
      |     data[1]=(GpsHomePos[1]*1e-7-116.2593683)/180*PIR*6362000+(double)st.localPos[1];
      |     data[2]=-GpsHomePos[2]*1e-3+(double)st.localPos[2];
      | }
      | 
      | The above structure is
      | struct outHILStateData{ // mavlink data forward from Pixhawk
      |     uint32_t time_boot_ms; //Timestamp of the message
      |     uint32_t copterID;     //Copter ID start from 1
      |     int32_t GpsPos[3];     //Estimated GPS position，lat&long: deg*1e7, alt: m*1e3 and up is positive
      |     int32_t GpsVel[3];     //Estimated GPS velocity, NED, m/s*1e2->cm/s
      |     int32_t gpsHome[3];     //Home GPS position, lat&long: deg*1e7, alt: m*1e3 and up is positive
      |     int32_t relative_alt;  //alt: m*1e3 and up is positive
      |     int32_t hdg;           //Course angle, NED,deg*1000, 0~360
      |     int32_t satellites_visible; //GPS Raw data, sum of satellite
      |     int32_t fix_type;     //GPS Raw data, Fixed type, 3 for fixed (good precision)
      |     int32_t resrveInit;       //Int, reserve for the future use
      |     float AngEular[3];    //Estimated Euler angle, unit: rad/s
      |     float localPos[3];    //Estimated locoal position, NED, unit: m
      |     float localVel[3];    //Estimated locoal velocity, NED, unit: m/s
      |     float pos_horiz_accuracy;   //GPS horizontal accuracy, unit: m
      |     float pos_vert_accuracy; //GPS vertical accuracy, unit: m
      |     float resrveFloat;      //float,reserve for the future use
      | }
      mask TypeOptions mode: CopterRecA | CopterRecB
  CopterRecB : S-Function  FunctionName=UDPSwarmAPI  Parameters=port,num,modeValue,T,ip  SFunctionDeploymentMode=off  EnableBusSupport=off  mask(UDP Receive){ip=127.0.0.1, port=29000, num=24, mode=CopterRecB, T=-1, modeValue=0}
      mask prompts: ip "UDP IP Address"; port "UDP Port"; num "vehicle Number"; mode "UDP Mode"; T "Sample Time"
      mask help:
      | This block receives bytes from an UDP/IP connection.
      | The first parameter is the UDP port on the first CopterSim App
      | The second parameter is the total vehicle number
      | The third parameter is the data mode. check the help button for the definition
      mask init:
      | if strcmp(mode,'CopterRecA')
      |     modeValue = 0;
      | elseif strcmp(mode,'CopterRecB') 
      |     modeValue = 1;
      | else
      |     modeValue = 0;
      | end
      mask Help:
      | UDP mode = 0 (localhost) or 1(broadcast), the 28-D output is defined as:
      | for(int i=0;i<3;i++){
      |     data[0+i]=(double)stl.gpsHome[i];
      |     data[3+i]=(double)stl.AngEular[i];
      |     data[6+i]=(double)stl.localPos[i];
      |     data[9+i]=(double)stl.localVel[i];
      |     data[12+i]=(double)stl.GpsPos[i];
      |     data[15+i]=(double)stl.GpsVel[i];
      | }
      | data[18] = (double)stl.time_boot_ms;
      | data[19] = (double)stl.copterID;
      | data[20] = (double)stl.relative_alt;
      | data[21] = (double)stl.hdg;
      | data[22] = (double)stl.satellites_visible;
      | data[23] = (double)stl.fix_type;
      | data[24] = (double)stl.resrveInit;
      | data[25] = (double)stl.pos_horiz_accuracy;
      | data[26] = (double)stl.pos_vert_accuracy;
      | data[27] = (double)stl.resrveFloat;
      | 
      | UDP mode =  2 (localhost) or 3(broadcast), 4,5 the 12-D output is defined as:
      | 
      | if(iUdpMode==2||iUdpMode==3){
      |     for(int i=0;i<3;i++){
      |         data[i]=(double)st.gpsHome[i];
      |         data[i+3]=(double)st.AngEular[i];
      |         data[i+6]=(double)st.localPos[i];
      |         data[i+9]=(double)st.localVel[i];
      |     }
      | }
      | if(iUdpMode==4||iUdpMode==5){
      |     double GpsHomePos[3];
      |     for(int i=0;i<3;i++){
      |             GpsHomePos[i] = (double)st.gpsHome[i];
      |             data[3+i]=(double)st.localPos[i];
      |             data[6+i]=(double)st.localVel[i];
      |             data[9+i]=(double)st.AngEular[i];
      |     }
      |     double PIR = 3.1415926536;
      |     data[0]=(GpsHomePos[0]*1e-7-40.1540302)/180*PIR*6362000+(double)st.localPos[0];
      |     data[1]=(GpsHomePos[1]*1e-7-116.2593683)/180*PIR*6362000+(double)st.localPos[1];
      |     data[2]=-GpsHomePos[2]*1e-3+(double)st.localPos[2];
      | }
      | 
      | The above structure is
      | struct outHILStateData{ // mavlink data forward from Pixhawk
      |     uint32_t time_boot_ms; //Timestamp of the message
      |     uint32_t copterID;     //Copter ID start from 1
      |     int32_t GpsPos[3];     //Estimated GPS position，lat&long: deg*1e7, alt: m*1e3 and up is positive
      |     int32_t GpsVel[3];     //Estimated GPS velocity, NED, m/s*1e2->cm/s
      |     int32_t gpsHome[3];     //Home GPS position, lat&long: deg*1e7, alt: m*1e3 and up is positive
      |     int32_t relative_alt;  //alt: m*1e3 and up is positive
      |     int32_t hdg;           //Course angle, NED,deg*1000, 0~360
      |     int32_t satellites_visible; //GPS Raw data, sum of satellite
      |     int32_t fix_type;     //GPS Raw data, Fixed type, 3 for fixed (good precision)
      |     int32_t resrveInit;       //Int, reserve for the future use
      |     float AngEular[3];    //Estimated Euler angle, unit: rad/s
      |     float localPos[3];    //Estimated locoal position, NED, unit: m
      |     float localVel[3];    //Estimated locoal velocity, NED, unit: m/s
      |     float pos_horiz_accuracy;   //GPS horizontal accuracy, unit: m
      |     float pos_vert_accuracy; //GPS vertical accuracy, unit: m
      |     float resrveFloat;      //float,reserve for the future use
      | }
      mask TypeOptions mode: CopterRecA | CopterRecB
  Demux{,1..19} (20 alike) : Demux  Outputs=21
  Display{1..3,5..6} (5 alike) : Display
  Mux{,2,4,6,8,10,12,14,16,18,20,22,24,26,28,30,32,34,36,38} (20 alike) : Mux  Inputs=3
  Mux{1,3,5,7,9,11,13,15,17,19,21,23,25,27,29,31,33,35,37,39} (20 alike) : Mux  Inputs=12
  Mux{40..49,51..60} (20 alike) : Mux  Inputs=2
  Mux50 : Mux  Inputs=20
  Out1 : Outport  VectorParamsAs1DForOutWhenUnconnected=off
  tag scope: battery_10=global, battery_11=global, battery_12=global, battery_13=global, battery_14=global, battery_15=global, battery_16=global, battery_17=global, battery_18=global, battery_19=global, battery_1=global, battery_20=global, battery_21=global, battery_22=global, battery_23=global, battery_24=global, battery_2=global, battery_3=global, battery_4=global, battery_5=global, battery_6=global, battery_7=global, battery_8=global, battery_9=global, copterRev10=global, copterRev11=global, copterRev12=global, copterRev13=global, copterRev14=global, copterRev15=global, copterRev16=global, copterRev17=global, copterRev18=global, copterRev19=global, copterRev1=global, copterRev20=global, copterRev2=global, copterRev3=global, copterRev4=global, copterRev5=global, copterRev6=global, copterRev7=global, copterRev8=global, copterRev9=global
  wires:
  [copterSend10] -> CopterRecA/10
  [copterSend6] -> CopterRecA/6
  CopterRecA/2 -> Demux1/1
  [copterSend4] -> CopterRecA/4
  [copterSend8] -> CopterRecA/8
  CopterRecA/1 -> Demux/1
  [copterSend5] -> CopterRecA/5
  [copterSend7] -> CopterRecA/7
  [copterSend9] -> CopterRecA/9
  [copterSend1] -> Display5/1, CopterRecA/1
  [copterSend2] -> CopterRecA/2
  [copterSend3] -> CopterRecA/3
  CopterRecB/22 -> [battery_22]
  CopterRecB/23 -> [battery_23]
  CopterRecB/24 -> Display3/1, [battery_24]
  CopterRecB/21 -> [battery_21]
  Demux/1 -> Mux/1
  Demux/2 -> Mux/2
  Demux/3 -> Mux/3
  Mux1/1 -> Display1/1, [copterRev1]
  Mux/1 -> [battery_1]
  Mux2/1 -> [battery_2]
  Mux3/1 -> [copterRev2]
  Mux4/1 -> [battery_3]
  Mux5/1 -> [copterRev3]
  CopterRecA/3 -> Demux2/1
  Mux6/1 -> [battery_4]
  Mux7/1 -> [copterRev4]
  CopterRecA/4 -> Demux3/1
  CopterRecA/5 -> Demux4/1
  CopterRecA/6 -> Demux5/1
  Mux12/1 -> [battery_7]
  Mux13/1 -> [copterRev7]
  Mux14/1 -> [battery_8]
  Mux15/1 -> [copterRev8]
  Mux16/1 -> [battery_9]
  Mux17/1 -> [copterRev9]
  Mux18/1 -> [battery_10]
  Mux19/1 -> [copterRev10]
  CopterRecA/10 -> Demux9/1
  Demux/4 -> Mux1/1
  Demux/5 -> Mux1/2
  Demux/6 -> Mux1/3
  Demux/7 -> Mux1/4
  Demux/8 -> Mux1/5
  Demux/9 -> Mux1/6
  Demux/10 -> Mux1/7
  Demux/11 -> Mux1/8
  Demux/12 -> Mux1/9
  Demux/13 -> Mux1/10
  Demux/14 -> Mux1/11
  Demux/15 -> Mux1/12
  Demux/20 -> Mux40/1
  Demux/21 -> Mux40/2
  [carSend7] -> CopterRecA1/7
  [carSend8] -> CopterRecA1/8
  [carSend5] -> CopterRecA1/5
  [carSend4] -> CopterRecA1/4
  [carSend6] -> CopterRecA1/6
  [carSend2] -> CopterRecA1/2
  [carSend10] -> CopterRecA1/10
  [carSend9] -> CopterRecA1/9
  [carSend3] -> CopterRecA1/3
  Mux35/1 -> [copterRev13]
  Mux28/1 -> [battery_19]
  Demux10/11 -> Mux21/8
  Mux30/1 -> [battery_20]
  Mux22/1 -> [battery_16]
  CopterRecA1/7 -> Demux16/1
  CopterRecA1/6 -> Demux15/1
  CopterRecA1/4 -> Demux13/1
  Demux10/5 -> Mux21/2
  Mux20/1 -> [battery_11]
  CopterRecA1/1 -> Demux10/1
  Demux10/4 -> Mux21/1
  Mux21/1 -> Display2/1, [copterRev11]
  Demux10/1 -> Mux20/1
  Demux10/2 -> Mux20/2
  Demux10/3 -> Mux20/3
  Mux31/1 -> [copterRev20]
  Demux10/14 -> Mux21/11
  Demux10/6 -> Mux21/3
  Demux10/7 -> Mux21/4
  CopterRecA1/5 -> Demux14/1
  Mux34/1 -> [battery_13]
  Mux26/1 -> [battery_18]
  CopterRecA1/3 -> Demux12/1
  Demux10/10 -> Mux21/7
  Mux23/1 -> [copterRev16]
  CopterRecA1/2 -> Demux11/1
  Demux10/8 -> Mux21/5
  Demux10/12 -> Mux21/9
  Demux10/15 -> Mux21/12
  Mux29/1 -> [copterRev19]
  Demux10/13 -> Mux21/10
  Mux39/1 -> [copterRev15]
  Demux10/9 -> Mux21/6
  CopterRecA1/8 -> Demux17/1
  CopterRecA1/10 -> Demux19/1
  Mux27/1 -> [copterRev18]
  Mux38/1 -> [battery_15]
  Demux1/1 -> Mux2/1
  Demux1/4 -> Mux3/1
  Demux1/10 -> Mux3/7
  Demux1/2 -> Mux2/2
  Demux1/6 -> Mux3/3
  Demux1/9 -> Mux3/6
  Demux1/14 -> Mux3/11
  Demux1/8 -> Mux3/5
  Demux1/5 -> Mux3/2
  Demux1/3 -> Mux2/3
  Demux1/7 -> Mux3/4
  Demux1/20 -> Mux51/1
  Demux1/13 -> Mux3/10
  Demux1/11 -> Mux3/8
  Demux1/12 -> Mux3/9
  Demux1/15 -> Mux3/12
  Demux1/21 -> Mux51/2
  Demux2/1 -> Mux4/1
  Demux2/4 -> Mux5/1
  Demux2/10 -> Mux5/7
  Demux2/2 -> Mux4/2
  Demux2/6 -> Mux5/3
  Demux2/9 -> Mux5/6
  Demux2/14 -> Mux5/11
  Demux2/8 -> Mux5/5
  Demux2/5 -> Mux5/2
  Demux2/3 -> Mux4/3
  Demux2/7 -> Mux5/4
  Demux2/20 -> Mux41/1
  Demux2/13 -> Mux5/10
  Demux2/11 -> Mux5/8
  Demux2/12 -> Mux5/9
  Demux2/15 -> Mux5/12
  Demux2/21 -> Mux41/2
  Demux19/1 -> Mux30/1
  Demux19/4 -> Mux31/1
  Demux19/10 -> Mux31/7
  Demux19/2 -> Mux30/2
  Demux19/6 -> Mux31/3
  Demux19/9 -> Mux31/6
  Demux19/14 -> Mux31/11
  Demux19/8 -> Mux31/5
  Demux19/5 -> Mux31/2
  Demux19/3 -> Mux30/3
  Demux19/7 -> Mux31/4
  Demux19/20 -> Mux42/1
  Demux19/13 -> Mux31/10
  Demux19/11 -> Mux31/8
  Demux19/12 -> Mux31/9
  Demux19/15 -> Mux31/12
  Demux18/1 -> Mux28/1
  Demux18/4 -> Mux29/1
  Demux18/10 -> Mux29/7
  Demux18/2 -> Mux28/2
  Demux18/6 -> Mux29/3
  Demux18/9 -> Mux29/6
  Demux18/14 -> Mux29/11
  Demux18/8 -> Mux29/5
  Demux18/5 -> Mux29/2
  Demux18/3 -> Mux28/3
  Demux18/7 -> Mux29/4
  Demux18/20 -> Mux52/1
  Demux18/13 -> Mux29/10
  Demux18/11 -> Mux29/8
  Demux18/12 -> Mux29/9
  Demux18/15 -> Mux29/12
  CopterRecA1/9 -> Demux18/1
  Demux18/21 -> Mux52/2
  Demux17/1 -> Mux26/1
  Demux17/4 -> Mux27/1
  Demux17/10 -> Mux27/7
  Demux17/2 -> Mux26/2
  Demux17/6 -> Mux27/3
  Demux17/9 -> Mux27/6
  Demux17/14 -> Mux27/11
  Demux17/8 -> Mux27/5
  Demux17/5 -> Mux27/2
  Demux17/3 -> Mux26/3
  Demux17/7 -> Mux27/4
  Demux17/20 -> Mux53/1
  Demux17/13 -> Mux27/10
  Demux17/11 -> Mux27/8
  Demux17/12 -> Mux27/9
  Demux17/15 -> Mux27/12
  Demux17/21 -> Mux53/2
  Demux19/21 -> Mux42/2
  Demux16/1 -> Mux24/1
  Demux16/4 -> Mux25/1
  Demux16/10 -> Mux25/7
  Demux16/2 -> Mux24/2
  Demux16/6 -> Mux25/3
  Demux16/9 -> Mux25/6
  Demux16/14 -> Mux25/11
  Demux16/8 -> Mux25/5
  Demux16/5 -> Mux25/2
  Demux16/3 -> Mux24/3
  Demux16/7 -> Mux25/4
  Demux16/20 -> Mux54/1
  Demux16/13 -> Mux25/10
  Demux16/11 -> Mux25/8
  Demux16/12 -> Mux25/9
  Demux16/15 -> Mux25/12
  Mux24/1 -> [battery_17]
  Demux15/1 -> Mux22/1
  Demux15/4 -> Mux23/1
  Demux15/10 -> Mux23/7
  Demux15/2 -> Mux22/2
  Demux15/6 -> Mux23/3
  Demux15/9 -> Mux23/6
  Demux15/14 -> Mux23/11
  Demux15/8 -> Mux23/5
  Demux15/5 -> Mux23/2
  Demux15/3 -> Mux22/3
  Demux15/7 -> Mux23/4
  Demux15/20 -> Mux55/1
  Demux15/13 -> Mux23/10
  Demux15/11 -> Mux23/8
  Demux15/12 -> Mux23/9
  Demux15/15 -> Mux23/12
  Demux15/21 -> Mux55/2
  Demux14/1 -> Mux38/1
  Demux14/4 -> Mux39/1
  Demux14/10 -> Mux39/7
  Demux14/2 -> Mux38/2
  Demux14/6 -> Mux39/3
  Demux14/9 -> Mux39/6
  Demux14/14 -> Mux39/11
  Demux14/8 -> Mux39/5
  Demux14/5 -> Mux39/2
  Demux14/3 -> Mux38/3
  Demux14/7 -> Mux39/4
  Demux14/20 -> Mux56/1
  Demux14/13 -> Mux39/10
  Demux14/11 -> Mux39/8
  Demux14/12 -> Mux39/9
  Demux14/15 -> Mux39/12
  Demux14/21 -> Mux56/2
  Demux13/1 -> Mux36/1
  Demux13/4 -> Mux37/1
  Demux13/10 -> Mux37/7
  Demux13/2 -> Mux36/2
  Demux13/6 -> Mux37/3
  Demux13/9 -> Mux37/6
  Demux13/14 -> Mux37/11
  Demux13/8 -> Mux37/5
  Demux13/5 -> Mux37/2
  Demux13/3 -> Mux36/3
  Demux13/7 -> Mux37/4
  Demux13/20 -> Mux57/1
  Demux13/13 -> Mux37/10
  Demux13/11 -> Mux37/8
  Demux13/12 -> Mux37/9
  Demux13/15 -> Mux37/12
  Mux37/1 -> [copterRev14]
  Mux36/1 -> [battery_14]
  Demux13/21 -> Mux57/2
  Demux12/1 -> Mux34/1
  Demux12/4 -> Mux35/1
  Demux12/10 -> Mux35/7
  Demux12/2 -> Mux34/2
  Demux12/6 -> Mux35/3
  Demux12/9 -> Mux35/6
  Demux12/14 -> Mux35/11
  Demux12/8 -> Mux35/5
  Demux12/5 -> Mux35/2
  Demux12/3 -> Mux34/3
  Demux12/7 -> Mux35/4
  Demux12/20 -> Mux58/1
  Demux12/13 -> Mux35/10
  Demux12/11 -> Mux35/8
  Demux12/12 -> Mux35/9
  Demux12/15 -> Mux35/12
  Demux12/21 -> Mux58/2
  Demux11/1 -> Mux32/1
  Demux11/4 -> Mux33/1
  Demux11/10 -> Mux33/7
  Demux11/2 -> Mux32/2
  Demux11/6 -> Mux33/3
  Demux11/9 -> Mux33/6
  Demux11/14 -> Mux33/11
  Demux11/8 -> Mux33/5
  Demux11/5 -> Mux33/2
  Demux11/3 -> Mux32/3
  Demux11/7 -> Mux33/4
  Demux11/20 -> Mux59/1
  Demux11/13 -> Mux33/10
  Demux11/11 -> Mux33/8
  Demux11/12 -> Mux33/9
  Demux11/15 -> Mux33/12
  Mux32/1 -> [battery_12]
  Mux33/1 -> [copterRev12]
  Demux11/21 -> Mux59/2
  Demux9/1 -> Mux18/1
  Demux9/4 -> Mux19/1
  Demux9/10 -> Mux19/7
  Demux9/2 -> Mux18/2
  Demux9/6 -> Mux19/3
  Demux9/9 -> Mux19/6
  Demux9/14 -> Mux19/11
  Demux9/8 -> Mux19/5
  Demux9/5 -> Mux19/2
  Demux9/3 -> Mux18/3
  Demux9/7 -> Mux19/4
  Demux9/20 -> Mux49/1
  Demux9/13 -> Mux19/10
  Demux9/11 -> Mux19/8
  Demux9/12 -> Mux19/9
  Demux9/15 -> Mux19/12
  Demux9/21 -> Mux49/2
  Demux16/21 -> Mux54/2
  Mux25/1 -> [copterRev17]
  Demux10/21 -> Mux60/2
  Demux10/20 -> Mux60/1
  Demux8/8 -> Mux17/5
  Demux8/21 -> Mux48/2
  Demux8/15 -> Mux17/12
  Demux8/5 -> Mux17/2
  Demux8/14 -> Mux17/11
  Demux8/6 -> Mux17/3
  Demux8/7 -> Mux17/4
  Demux8/10 -> Mux17/7
  Demux8/4 -> Mux17/1
  Demux8/3 -> Mux16/3
  Demux8/13 -> Mux17/10
  Demux8/12 -> Mux17/9
  Demux8/11 -> Mux17/8
  Demux8/2 -> Mux16/2
  Demux8/9 -> Mux17/6
  Demux8/20 -> Mux48/1
  Demux8/1 -> Mux16/1
  Demux7/8 -> Mux15/5
  Demux7/21 -> Mux47/2
  Demux7/15 -> Mux15/12
  Demux7/5 -> Mux15/2
  Demux7/14 -> Mux15/11
  Demux7/6 -> Mux15/3
  Demux7/7 -> Mux15/4
  Demux7/10 -> Mux15/7
  Demux7/4 -> Mux15/1
  Demux7/3 -> Mux14/3
  Demux7/13 -> Mux15/10
  Demux7/12 -> Mux15/9
  Demux7/11 -> Mux15/8
  Demux7/2 -> Mux14/2
  Demux7/9 -> Mux15/6
  Demux7/20 -> Mux47/1
  Demux7/1 -> Mux14/1
  CopterRecA/8 -> Demux7/1
  Demux5/8 -> Mux11/5
  Demux5/21 -> Mux45/2
  Demux5/15 -> Mux11/12
  Demux5/5 -> Mux11/2
  Demux5/14 -> Mux11/11
  Demux5/6 -> Mux11/3
  Demux5/7 -> Mux11/4
  Demux5/10 -> Mux11/7
  Demux5/4 -> Mux11/1
  Demux5/3 -> Mux10/3
  Demux5/13 -> Mux11/10
  Demux5/12 -> Mux11/9
  Demux5/11 -> Mux11/8
  Demux5/2 -> Mux10/2
  Demux5/9 -> Mux11/6
  Demux5/20 -> Mux45/1
  Demux5/1 -> Mux10/1
  Mux10/1 -> [battery_6]
  Mux11/1 -> [copterRev6]
  Demux4/8 -> Mux9/5
  Demux4/21 -> Mux44/2
  Demux4/15 -> Mux9/12
  Demux4/5 -> Mux9/2
  Demux4/14 -> Mux9/11
  Demux4/6 -> Mux9/3
  Demux4/7 -> Mux9/4
  Demux4/10 -> Mux9/7
  Demux4/4 -> Mux9/1
  Demux4/3 -> Mux8/3
  Demux4/13 -> Mux9/10
  Demux4/12 -> Mux9/9
  Demux4/11 -> Mux9/8
  Demux4/2 -> Mux8/2
  Demux4/9 -> Mux9/6
  Demux4/20 -> Mux44/1
  Demux4/1 -> Mux8/1
  Mux9/1 -> [copterRev5]
  Demux6/8 -> Mux13/5
  Demux6/21 -> Mux46/2
  Demux6/15 -> Mux13/12
  Demux6/5 -> Mux13/2
  Demux6/14 -> Mux13/11
  Demux6/6 -> Mux13/3
  Demux6/7 -> Mux13/4
  Demux6/10 -> Mux13/7
  Demux6/4 -> Mux13/1
  Demux6/3 -> Mux12/3
  Demux6/13 -> Mux13/10
  Demux6/12 -> Mux13/9
  Demux6/11 -> Mux13/8
  Demux6/2 -> Mux12/2
  Demux6/9 -> Mux13/6
  Demux6/20 -> Mux46/1
  Demux6/1 -> Mux12/1
  CopterRecA/7 -> Demux6/1
  Mux8/1 -> [battery_5]
  Demux3/8 -> Mux7/5
  Demux3/21 -> Mux43/2
  Demux3/15 -> Mux7/12
  Demux3/5 -> Mux7/2
  Demux3/14 -> Mux7/11
  Demux3/6 -> Mux7/3
  Demux3/7 -> Mux7/4
  Demux3/10 -> Mux7/7
  Demux3/4 -> Mux7/1
  Demux3/3 -> Mux6/3
  Demux3/13 -> Mux7/10
  Demux3/12 -> Mux7/9
  Demux3/11 -> Mux7/8
  Demux3/2 -> Mux6/2
  Demux3/9 -> Mux7/6
  Demux3/20 -> Mux43/1
  Demux3/1 -> Mux6/1
  CopterRecA/9 -> Demux8/1
  Mux50/1 -> Out1/1
  Mux40/1 -> Mux50/1
  Mux51/1 -> Mux50/2
  Mux41/1 -> Mux50/3
  Mux43/1 -> Mux50/4
  Mux44/1 -> Mux50/5
  Mux45/1 -> Mux50/6
  Mux46/1 -> Mux50/7
  Mux47/1 -> Mux50/8
  Mux48/1 -> Mux50/9
  Mux49/1 -> Mux50/10
  Mux60/1 -> Mux50/11
  Mux59/1 -> Mux50/12
  Mux58/1 -> Mux50/13
  Mux57/1 -> Mux50/14
  Mux56/1 -> Mux50/15
  Mux55/1 -> Mux50/16
  Mux54/1 -> Mux50/17
  Mux53/1 -> Mux50/18
  Mux52/1 -> Mux50/19
  Mux42/1 -> Mux50/20
  [carSend1] -> CopterRecA1/1, Display6/1
